simulink model "A6_PID_control"  (R2023a)
settings: Solver=FixedStepAuto  StartTime=0.0  StopTime=20  FixedStep=0.01  RelTol=1e-3
values from neighbouring files (symbols this model uses):
  CAf = 1.0    (= 1)    [A1_find_steady_state.m]    (also in A2_Task9_param_consts.m)
  Cp = 0.239    [A1_find_steady_state.m]    (also in A2_Task9_param_consts.m)
  dHr = -5e4    (= -50000)    [A1_find_steady_state.m]    (also in A2_Task9_param_consts.m)
  ER = 8750    [A1_find_steady_state.m]    (also in A2_Task9_param_consts.m)
  k0 = 6.379829e10    (= 63798290000)    [A1_find_steady_state.m]    (also in A2_Task9_param_consts.m)
  q = 100    [A1_find_steady_state.m]    (also in A2_Task9_param_consts.m)
  rho = 1000    [A1_find_steady_state.m]    (also in A2_Task9_param_consts.m)
  Tf = 350    [A1_find_steady_state.m]    (also in A2_Task9_param_consts.m)
  UA = 5e4    (= 50000)    [A1_find_steady_state.m]    (also in A2_Task9_param_consts.m)
  V = 100    [A1_find_steady_state.m]    (also in A2_Task9_param_consts.m)
libraries: slpidlib x1
settings Model: Creator=xiong  LastModifiedBy=xiong

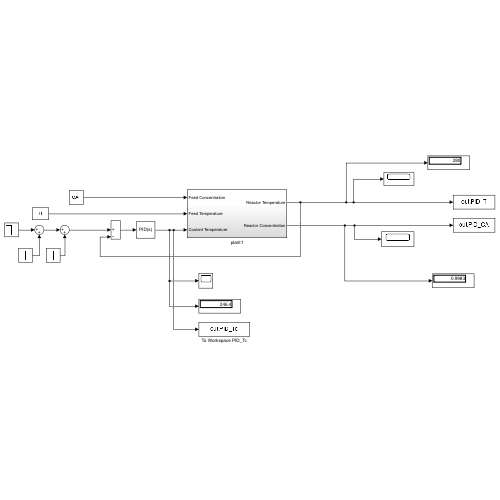
[thumbnail: Simulink's stored preview of the top-level diagram]
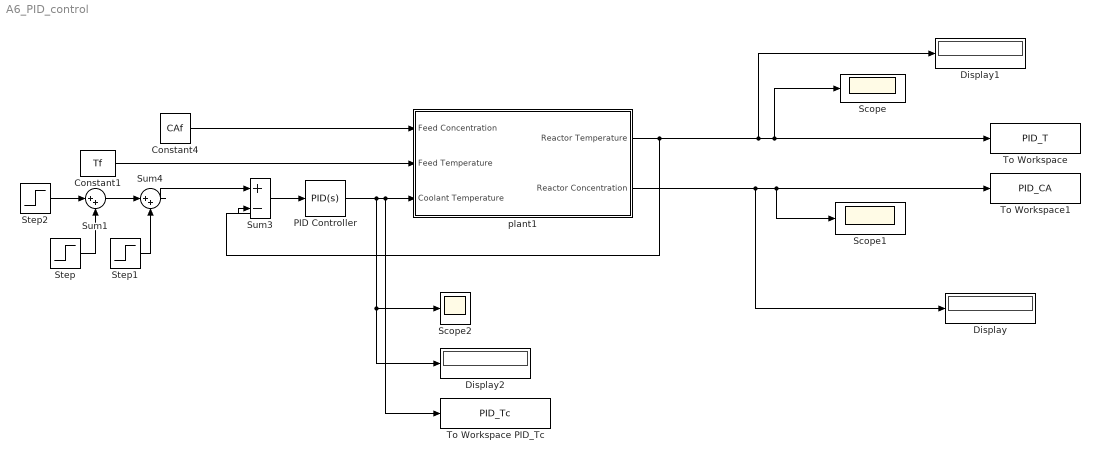
== system A6_PID_control ==
  Constant1 : Constant  Value=Tf
  Constant4 : Constant  Value=CAf
  Display : Display
  Display1 : Display
  Display2 : Display
  PID Controller : slpidlib/PID Controller  Controller=PID  Form=Parallel  TimeDomain=Continuous-time  UseExternalTs=off  SampleTime=-1  IntegratorMethod=Forward Euler  FilterMethod=Forward Euler  ControllerParametersSource=internal  P=53.775  I=3220  UseKiTs=off  D=0  N=0  UseFilter=on  TunerSelectOption=Transfer Function Based (PID Tuner App)  InitialConditionSource=internal  InitialConditionForIntegrator=0  InitialConditionForFilter=0  DifferentiatorICPrevScaledInput=0  ExternalReset=none  TrackingMode=off  Kt=1  LimitOutput=off  SatLimitsSource=internal  UpperSaturationLimit=inf  LowerSaturationLimit=-inf  LinearizeAsGain=on  AntiWindupMode=none  Kb=1  LimitIntegrator=off  UpperIntegratorSaturationLimit=inf  LowerIntegratorSaturationLimit=-inf  POutMin=[]  POutMax=[]  IOutMin=[]  IOutMax=[]  DOutMin=[]  DOutMax=[]  NOutMin=[]  NOutMax=[]  SumOutMin=[]  SumOutMax=[]  SaturationOutMin=[]  SaturationOutMax=[]  PParamMin=[]  PParamMax=[]  IParamMin=[]  IParamMax=[]  DParamMin=[]  DParamMax=[]  NParamMin=[]  NParamMax=[]  KbParamMin=[]  KbParamMax=[]  KtParamMin=[]  KtParamMax=[]  KbOutMin=[]  KbOutMax=[]  KtOutMin=[]  KtOutMax=[]  IntegratorOutMin=[]  IntegratorOutMax=[]  FilterOutMin=[]  FilterOutMax=[]  SumI1OutMin=[]  SumI1OutMax=[]  SumI2OutMin=[]  SumI2OutMax=[]  SumI3OutMin=[]  SumI3OutMax=[]  SumI4OutMin=[]  SumI4OutMax=[]  SumDOutMin=[]  SumDOutMax=[]  DifferentiatorOutMin=[]  DifferentiatorOutMax=[]  FilterDiffOutCoefMin=[]  FilterDiffOutCoefMax=[]  ReciprocalOutMin=[]  ReciprocalOutMax=[]  SumDenOutMin=[]  SumDenOutMax=[]  SumNumOutMin=[]  SumNumOutMax=[]  DivideOutMin=[]  DivideOutMax=[]  UdiffTsProdOutMin=[]  UdiffTsProdOutMax=[]  NTsProdOutMin=[]  NTsProdOutMax=[]  UintegralTsProdOutMin=[]  UintegralTsProdOutMax=[]  UngainTsProdOutMin=[]  UngainTsProdOutMax=[]  ClampingZeroOutDataTypeStr=Inherit: Inherit via back propagation  ClampingZeroOutMin=[]  ClampingZeroOutMax=[]  FilterDenConstantOutDataTypeStr=Inherit: Inherit via back propagation  FilterDenConstantOutMin=[]  FilterDenConstantOutMax=[]  PCopyOutDataTypeStr=Inherit: Inherit via back propagation  PCopyOutMin=[]  PCopyOutMax=[]  NCopyOutDataTypeStr=Inherit: Inherit via back propagation  NCopyOutMin=[]  NCopyOutMax=[]  IntegratorContinuousStateAttributes=''  IntegratorStateMustResolveToSignalObject=off  IntegratorRTWStateStorageClass=Auto  FilterContinuousStateAttributes=''  FilterStateMustResolveToSignalObject=off  FilterRTWStateStorageClass=Auto  ParallelPVariant=InternalParameters  IdealPVariant=Disabled  IVariant=InternalParameters  DVariant=InternalParameters  IntegratorVariant=Continuous  SatVariant=Disabled  AWVariant=Passthrough  PCopyVariant=Disabled  TRVariant=Disabled  FdbkBlocksVariant=Forward  IdealPFdbkVariant=Disabled  SatFdbkVariant=Disabled  DerivativeFilterVariant=ContFilter  NVariant=InternalParameters  NCopyVariant=Disabled  FilterICVariant=InternalICsFilter  IntegratorICVariant=InternalICs  ExternalResetVariant=Disabled  TRSumVariant=Passthrough  SumFdbkVariant=Disabled  SumVariant=Sum_PID  TsampFilterVariant=InternalTs  TsampNgainVariant=Passthrough  TsampIntegralVariant=Disabled_SignalSpec  ExternalSaturationOutDataTypeStr=Inherit: Same as second input
  Scope : Scope
  Scope1 : Scope
  Scope2 : Scope
  Step : Step  Time=8  After=20  SampleTime=0.1
  Step1 : Step  Time=12  After=-40  SampleTime=0.1
  Step2 : Step  Time=4  Before=303  After=300  SampleTime=0.1
  Sum1 : Sum  Inputs=|++
  Sum3 : Sum  Inputs=|+-
  Sum4 : Sum  Inputs=|++
  To Workspace : ToWorkspace  VariableName=PID_T  SaveFormat=Timeseries  SampleTime=-1
  To Workspace PID_Tc : ToWorkspace  VariableName=PID_Tc  SaveFormat=Timeseries  SampleTime=-1
  To Workspace1 : ToWorkspace  VariableName=PID_CA  SaveFormat=Timeseries  SampleTime=-1
  plant1 : Subsystem
  wires:
  plant1/1(Reactor Temperature) -> Sum3/2, Display1/1, To Workspace/1, Scope/1
  Step2/1 -> Sum1/1
  plant1/2(Reactor Concentration) -> To Workspace1/1, Scope1/1, Display/1
  Constant4/1 -> plant1/1(Feed Concentration)
  Constant1/1 -> plant1/2(Feed Temperature)
  Sum1/1 -> Sum4/1
  Step/1 -> Sum1/2
  Step1/1 -> Sum4/2
  Sum4/1 -> Sum3/1
  Sum3/1 -> PID Controller/1
  PID Controller/1 -> To Workspace PID_Tc/1, plant1/3(Coolant Temperature), Display2/1, Scope2/1

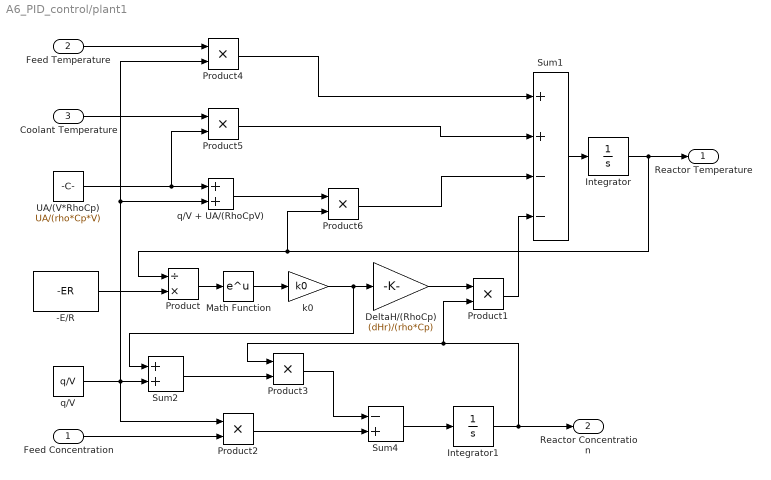
== system A6_PID_control/plant1 ==
  Feed Concentration : Inport
  Feed Temperature : Inport  Port=2
  Coolant Temperature : Inport  Port=3
  -E/R : Constant  Value=-ER
  DeltaH/(RhoCp) : Gain  Gain=(dHr)/(rho*Cp)  SaturateOnIntegerOverflow=on  OutDataTypeStr=Inherit: Same as input  ParamDataTypeStr=Inherit: Same as input
  Integrator : Integrator  InitialCondition=303.49  LimitOutput=on  LowerSaturationLimit=0
  Integrator1 : Integrator  InitialCondition=0.9803  LimitOutput=on  LowerSaturationLimit=0
  Math Function : Math  SignedPower=on
  Product : Product  Inputs=/*  InputSameDT=on  RndMeth=Zero  SaturateOnIntegerOverflow=on  OutDataTypeStr=Inherit: Same as first input
  Product1 : Product  InputSameDT=on  RndMeth=Zero  SaturateOnIntegerOverflow=on  OutDataTypeStr=Inherit: Same as first input
  Product{2,4..6} (4 alike) : Product
  Product3 : Product  InputSameDT=on  RndMeth=Zero  SaturateOnIntegerOverflow=on  OutDataTypeStr=Inherit: Same as first input
  Sum1 : Sum  Inputs=++--  InputSameDT=on  SaturateOnIntegerOverflow=on  OutDataTypeStr=Inherit: Same as first input
  Sum2 : Sum  InputSameDT=on  SaturateOnIntegerOverflow=on  OutDataTypeStr=Inherit: Same as first input
  Sum4 : Sum  Inputs=-+  InputSameDT=on  SaturateOnIntegerOverflow=on  OutDataTypeStr=Inherit: Same as first input
  UA/(V*RhoCp) : Constant  Value=UA/(rho*Cp*V)
  k0 : Gain  Gain=k0  SaturateOnIntegerOverflow=on  OutDataTypeStr=Inherit: Same as input  ParamDataTypeStr=Inherit: Same as input
  q/V : Constant  Value=q/V
  q/V + UA/(RhoCpV) : Sum
  Reactor Temperature : Outport
  Reactor Concentration : Outport  Port=2
  wires:
  Product4/1 -> Sum1/1
  Sum1/1 -> Integrator/1
  Integrator/1 -> Product6/2, Product/1, Reactor Temperature/1
  Product5/1 -> Sum1/2
  Product6/1 -> Sum1/3
  Product/1 -> Math Function/1
  Math Function/1 -> k0/1
  DeltaH/(RhoCp)/1 -> Product1/1
  Product1/1 -> Sum1/4
  k0/1 -> DeltaH/(RhoCp)/1, Sum2/1
  -E/R/1 -> Product/2
  Product3/1 -> Sum4/1
  Sum4/1 -> Integrator1/1
  Integrator1/1 -> Product1/2, Product3/1, Reactor Concentration/1
  q/V/1 -> Product2/1, Sum2/2, Product4/2, q/V + UA/(RhoCpV)/2
  Product2/1 -> Sum4/2
  Feed Temperature/1 -> Product4/1
  Feed Concentration/1 -> Product2/2
  Coolant Temperature/1 -> Product5/1
  Sum2/1 -> Product3/2
  UA/(V*RhoCp)/1 -> Product5/2, q/V + UA/(RhoCpV)/1
  q/V + UA/(RhoCpV)/1 -> Product6/1
